simulink model "MQTT_pubsub"  (R2017b)
settings: Solver=FixedStepDiscrete  StartTime=0.0  StopTime=10.0  FixedStep=1e-3  RelTol=1e-3
libraries: mbed_ethernet_mqtt x3, mbed_lib x2, mbed_ethernet x1
settings Model: Creator=oh  LastModifiedBy=oh
settings OptimizationCC: DefaultParameterBehavior=Inlined  PassReuseOutputArgsAs=Individual arguments
settings DebuggingCC: ParameterTunabilityLossMsg=error
settings HardwareCC: ProdBitPerPointer=32  ProdBitPerSizeT=32  ProdBitPerPtrDiffT=32  ProdLargestAtomicInteger=Long  ProdLargestAtomicFloat=Double  ProdWordSize=32  ProdHWDeviceType=ARM Compatible->ARM Cortex
settings SFSimCC: MATLABDynamicMemAlloc=off
settings RTWCC: SystemTargetFile=mbed.tlc  TemplateMakefile=mbed.tmf  Description=MbedTarget (Embedded Target for Embedded Coder)  IncludeHyperlinkInReport=on  TargetLang=C++
settings CodeAppCC: ForceParamTrailComments=on  IgnoreCustomStorageClasses=off  OperatorAnnotations=on  SimulinkDataObjDesc=on  SFDataObjDesc=on  InsertBlockDesc=on
settings STFCustomTargetCC: TargetLibSuffix=.a  TargetLangStandard=C++03 (ISO)  MultiwordLength=256  GenerateSampleERTMain=on  CombineOutputUpdateFcns=on  ERTCustomFileBanners=on  SupportContinuousTime=off  SupportNonInlinedSFcns=off  RemoveResetFunc=on  MATLABClassNameForMDSCustomization=Simulink.SoftwareTarget.ERTCustomization  ModelStepFunctionPrototypeControlCompliant=on  GRTInterface=off  SystemTargetFile=mbed.tlc
settings ERTTargetCC: TargetLangStandard=C++03 (ISO)  GenerateSampleERTMain=on  ParMdlRefBuildCompliant=off  CompOptLevelCompliant=off  ConcurrentExecutionCompliant=off  CPPClassGenCompliant=off  UseToolchainInfoCompliant=off  InlinedParameterPlacement=NonHierarchical  ERTCustomFileTemplate=mbed_file_process.tlc

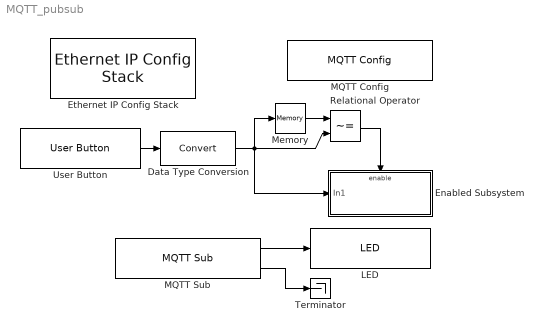
== system MQTT_pubsub ==
  Data Type Conversion : DataTypeConversion
  Enabled Subsystem : Subsystem  TreatAsAtomicUnit=on
  Ethernet IP Config Stack : mbed_ethernet/Ethernet IP Config Stack  Priority=0  sDHCP=on  DHCP=1  ip_addr=192.168.178.25  sub_mask=255.255.255.0  gateway=192.168.178.1  SerialDebugInfo=on
      settings: SourceProductName=Mbed Target
  LED : mbed_lib/GPIO/LED  nLED=1  SampleTime=-1
      settings: SourceProductName=Mbed Target
  MQTT Config : mbed_ethernet_mqtt/MQTT Config  Priority=0  broker_ip=192.168.178.25  broker_port=1883
      settings: SourceProductName=Mbed Target
  MQTT Sub : mbed_ethernet_mqtt/MQTT Sub  Priority=1  MQTT_topic=test/topic/led  BufferSize=1  SampleTime=0.01
      settings: SourceProductName=Mbed Target
  Memory : Memory
  Relational Operator : RelationalOperator  Operator=~=  OutDataTypeStr=boolean  RndMeth=Simplest
  Terminator : Terminator
  User Button : mbed_lib/GPIO/User Button  SampleTime=1
      settings: SourceProductName=Mbed Target
  wires:
  User Button/1 -> Data Type Conversion/1
  Data Type Conversion/1 -> Memory/1, Relational Operator/2, Enabled Subsystem/1(In1)
  MQTT Sub/1 -> LED/1
  MQTT Sub/2 -> Terminator/1
  Memory/1 -> Relational Operator/1
  Relational Operator/1 -> Enabled Subsystem/Enable

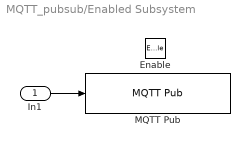
== system MQTT_pubsub/Enabled Subsystem ==
  In1 : Inport
  Enable : EnablePort
  MQTT Pub : mbed_ethernet_mqtt/MQTT Pub  Priority=2  MQTT_topic=test/topic/button  BufferSize=100  numData=off  SampleTime=-1
      settings: SourceProductName=Mbed Target
  wires:
  In1/1 -> MQTT Pub/1
